simulink model "Par2_1"  (R2018a)
settings: Solver=VariableStepAuto  StartTime=0.0  StopTime=100  RelTol=1e-3
settings Model: Creator=wangluo  LastModifiedBy=wangluo

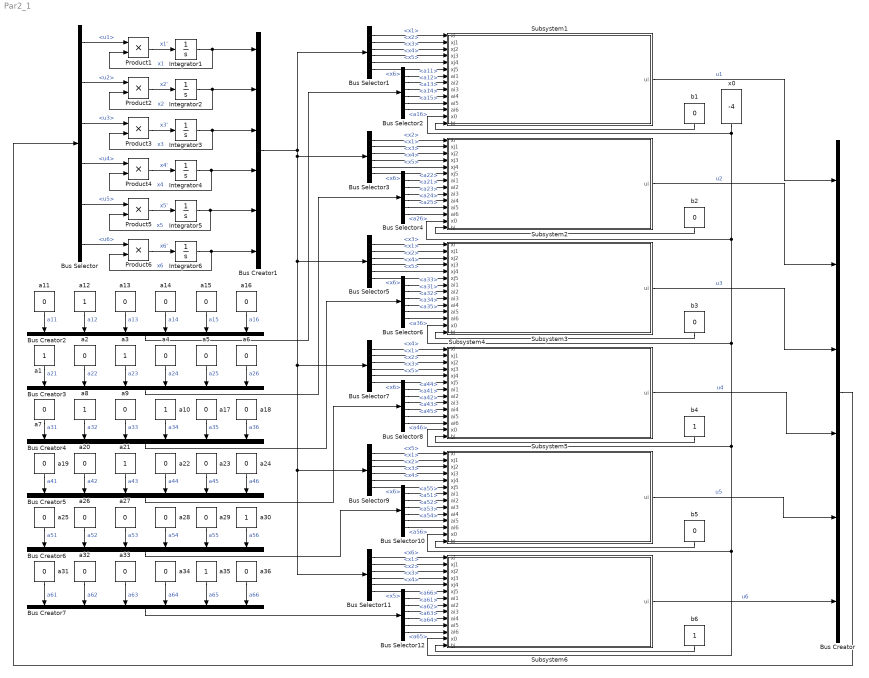
== system Par2_1 ==
  Bus Creator{,1..7} (8 alike) : BusCreator  Inputs=6
  Bus Selector : BusSelector  OutputSignals=u1,u2,u3,u4,u5,u6
  Bus Selector1 : BusSelector  OutputSignals=x1,x2,x3,x4,x5,x6
  Bus Selector10 : BusSelector  OutputSignals=a55,a51,a52,a53,a54,a56
  Bus Selector11 : BusSelector  OutputSignals=x6,x1,x2,x3,x4,x5
  Bus Selector12 : BusSelector  OutputSignals=a66,a61,a62,a63,a64,a65
  Bus Selector2 : BusSelector  OutputSignals=a11,a12,a13,a14,a15,a16
  Bus Selector3 : BusSelector  OutputSignals=x2,x1,x3,x4,x5,x6
  Bus Selector4 : BusSelector  OutputSignals=a22,a21,a23,a24,a25,a26
  Bus Selector5 : BusSelector  OutputSignals=x3,x1,x2,x4,x5,x6
  Bus Selector6 : BusSelector  OutputSignals=a33,a31,a32,a34,a35,a36
  Bus Selector7 : BusSelector  OutputSignals=x4,x1,x2,x3,x5,x6
  Bus Selector8 : BusSelector  OutputSignals=a44,a41,a42,a43,a45,a46
  Bus Selector9 : BusSelector  OutputSignals=x5,x1,x2,x3,x4,x6
  Integrator1 : Integrator  InitialCondition=1
  Integrator2 : Integrator  InitialCondition=7
  Integrator3 : Integrator  InitialCondition=0.5
  Integrator4 : Integrator  InitialCondition=5
  Integrator5 : Integrator  InitialCondition=3
  Integrator6 : Integrator  InitialCondition=8
  Product{1..6} (6 alike) : Product
  Subsystem1 : Subsystem
  Subsystem2 : Subsystem
  Subsystem3 : Subsystem
  Subsystem4 : Subsystem
  Subsystem5 : Subsystem
  Subsystem6 : Subsystem
  a{1,3,8,10,12,21,30,35} (8 alike) : Constant
  a{2,4..7,9,11,13..20,22..29,31..34,36} (28 alike) : Constant  Value=0
  b{1..3,5} (4 alike) : Constant  Value=0
  b4 : Constant
  b6 : Constant
  x0 : Constant  Value=-4
  wires:
  Integrator1/1 -> Product1/2, Bus Creator1/1  "x1"
  Integrator2/1 -> Product2/2, Bus Creator1/2  "x2"
  Bus Creator/1 -> Bus Selector/1
  Subsystem2/1(ui) -> Bus Creator/2  "u2"
  Subsystem3/1(ui) -> Bus Creator/3  "u3"
  Subsystem4/1(ui) -> Bus Creator/4  "u4"
  Subsystem5/1(ui) -> Bus Creator/5  "u5"
  Subsystem6/1(ui) -> Bus Creator/6  "u6"
  Product1/1 -> Integrator1/1  "x1'"
  Product4/1 -> Integrator4/1  "x4'"
  Product3/1 -> Integrator3/1  "x3'"
  Product2/1 -> Integrator2/1  "x2'"
  Product5/1 -> Integrator5/1  "x5'"
  Product6/1 -> Integrator6/1  "x6'"
  Integrator3/1 -> Product3/2, Bus Creator1/3  "x3"
  Integrator4/1 -> Product4/2, Bus Creator1/4  "x4"
  Integrator5/1 -> Product5/2, Bus Creator1/5  "x5"
  Integrator6/1 -> Product6/2, Bus Creator1/6  "x6"
  Bus Selector/3 -> Product3/1  "<u3>"
  Bus Selector/1 -> Product1/1  "<u1>"
  Bus Selector/2 -> Product2/1  "<u2>"
  Bus Selector/4 -> Product4/1  "<u4>"
  Bus Selector/5 -> Product5/1  "<u5>"
  Bus Selector/6 -> Product6/1  "<u6>"
  Bus Selector1/1 -> Subsystem1/1(xi)  "<x1>"
  Bus Selector1/2 -> Subsystem1/2(xj1)  "<x2>"
  Bus Selector1/3 -> Subsystem1/3(xj2)  "<x3>"
  Bus Selector1/4 -> Subsystem1/4(xj3)  "<x4>"
  Bus Selector1/5 -> Subsystem1/5(xj4)  "<x5>"
  Bus Selector1/6 -> Subsystem1/6(xj5)  "<x6>"
  Bus Creator1/1 -> Bus Selector3/1, Bus Selector5/1, Bus Selector11/1, Bus Selector9/1, Bus Selector7/1, Bus Selector1/1
  a13/1 -> Bus Creator2/3  "a13"
  a14/1 -> Bus Creator2/4  "a14"
  a11/1 -> Bus Creator2/1  "a11"
  a12/1 -> Bus Creator2/2  "a12"
  a15/1 -> Bus Creator2/5  "a15"
  a16/1 -> Bus Creator2/6  "a16"
  Bus Creator2/1 -> Bus Selector2/1
  a4/1 -> Bus Creator3/4  "a24"
  a6/1 -> Bus Creator3/6  "a26"
  Bus Creator3/1 -> Bus Selector4/1
  a5/1 -> Bus Creator3/5  "a25"
  a3/1 -> Bus Creator3/3  "a23"
  a2/1 -> Bus Creator3/2  "a22"
  a1/1 -> Bus Creator3/1  "a21"
  a10/1 -> Bus Creator4/4  "a34"
  a18/1 -> Bus Creator4/6  "a36"
  Bus Creator4/1 -> Bus Selector6/1
  a17/1 -> Bus Creator4/5  "a35"
  a9/1 -> Bus Creator4/3  "a33"
  a8/1 -> Bus Creator4/2  "a32"
  a7/1 -> Bus Creator4/1  "a31"
  a22/1 -> Bus Creator5/4  "a44"
  a24/1 -> Bus Creator5/6  "a46"
  Bus Creator5/1 -> Bus Selector8/1
  a23/1 -> Bus Creator5/5  "a45"
  a21/1 -> Bus Creator5/3  "a43"
  a20/1 -> Bus Creator5/2  "a42"
  a19/1 -> Bus Creator5/1  "a41"
  a28/1 -> Bus Creator6/4  "a54"
  a30/1 -> Bus Creator6/6  "a56"
  Bus Creator6/1 -> Bus Selector10/1
  a29/1 -> Bus Creator6/5  "a55"
  a27/1 -> Bus Creator6/3  "a53"
  a26/1 -> Bus Creator6/2  "a52"
  a25/1 -> Bus Creator6/1  "a51"
  a34/1 -> Bus Creator7/4  "a64"
  a36/1 -> Bus Creator7/6  "a66"
  Bus Creator7/1 -> Bus Selector12/1
  a35/1 -> Bus Creator7/5  "a65"
  a33/1 -> Bus Creator7/3  "a63"
  a32/1 -> Bus Creator7/2  "a62"
  a31/1 -> Bus Creator7/1  "a61"
  b1/1 -> Subsystem1/14(bi)
  b3/1 -> Subsystem3/14(bi)
  b4/1 -> Subsystem4/14(bi)
  b5/1 -> Subsystem5/14(bi)
  b6/1 -> Subsystem6/14(bi)
  x0/1 -> Subsystem2/13(x0), Subsystem3/13(x0), Subsystem6/13(x0), Subsystem5/13(x0), Subsystem4/13(x0), Subsystem1/13(x0)
  Subsystem1/1(ui) -> Bus Creator/1  "u1"
  Bus Selector3/1 -> Subsystem2/1(xi)  "<x2>"
  Bus Selector3/3 -> Subsystem2/3(xj2)  "<x3>"
  Bus Selector3/4 -> Subsystem2/4(xj3)  "<x4>"
  Bus Selector3/5 -> Subsystem2/5(xj4)  "<x5>"
  Bus Selector3/6 -> Subsystem2/6(xj5)  "<x6>"
  Bus Selector2/1 -> Subsystem1/7(ai1)  "<a11>"
  Bus Selector2/2 -> Subsystem1/8(ai2)  "<a12>"
  Bus Selector2/3 -> Subsystem1/9(ai3)  "<a13>"
  Bus Selector2/4 -> Subsystem1/10(ai4)  "<a14>"
  Bus Selector2/5 -> Subsystem1/11(ai5)  "<a15>"
  Bus Selector2/6 -> Subsystem1/12(ai6)  "<a16>"
  Bus Selector3/2 -> Subsystem2/2(xj1)  "<x1>"
  b2/1 -> Subsystem2/14(bi)
  Bus Selector5/1 -> Subsystem3/1(xi)  "<x3>"
  Bus Selector5/2 -> Subsystem3/2(xj1)  "<x1>"
  Bus Selector5/3 -> Subsystem3/3(xj2)  "<x2>"
  Bus Selector5/4 -> Subsystem3/4(xj3)  "<x4>"
  Bus Selector5/5 -> Subsystem3/5(xj4)  "<x5>"
  Bus Selector5/6 -> Subsystem3/6(xj5)  "<x6>"
  Bus Selector7/1 -> Subsystem4/1(xi)  "<x4>"
  Bus Selector7/2 -> Subsystem4/2(xj1)  "<x1>"
  Bus Selector7/3 -> Subsystem4/3(xj2)  "<x2>"
  Bus Selector7/4 -> Subsystem4/4(xj3)  "<x3>"
  Bus Selector7/5 -> Subsystem4/5(xj4)  "<x5>"
  Bus Selector7/6 -> Subsystem4/6(xj5)  "<x6>"
  Bus Selector4/1 -> Subsystem2/7(ai1)  "<a22>"
  Bus Selector4/2 -> Subsystem2/8(ai2)  "<a21>"
  Bus Selector4/3 -> Subsystem2/9(ai3)  "<a23>"
  Bus Selector4/4 -> Subsystem2/10(ai4)  "<a24>"
  Bus Selector4/5 -> Subsystem2/11(ai5)  "<a25>"
  Bus Selector4/6 -> Subsystem2/12(ai6)  "<a26>"
  Bus Selector6/1 -> Subsystem3/7(ai1)  "<a33>"
  Bus Selector6/2 -> Subsystem3/8(ai2)  "<a31>"
  Bus Selector6/3 -> Subsystem3/9(ai3)  "<a32>"
  Bus Selector6/4 -> Subsystem3/10(ai4)  "<a34>"
  Bus Selector6/5 -> Subsystem3/11(ai5)  "<a35>"
  Bus Selector6/6 -> Subsystem3/12(ai6)  "<a36>"
  Bus Selector8/1 -> Subsystem4/7(ai1)  "<a44>"
  Bus Selector8/2 -> Subsystem4/8(ai2)  "<a41>"
  Bus Selector8/3 -> Subsystem4/9(ai3)  "<a42>"
  Bus Selector8/4 -> Subsystem4/10(ai4)  "<a43>"
  Bus Selector8/5 -> Subsystem4/11(ai5)  "<a45>"
  Bus Selector8/6 -> Subsystem4/12(ai6)  "<a46>"
  Bus Selector9/1 -> Subsystem5/1(xi)  "<x5>"
  Bus Selector9/2 -> Subsystem5/2(xj1)  "<x1>"
  Bus Selector9/3 -> Subsystem5/3(xj2)  "<x2>"
  Bus Selector9/4 -> Subsystem5/4(xj3)  "<x3>"
  Bus Selector9/5 -> Subsystem5/5(xj4)  "<x4>"
  Bus Selector9/6 -> Subsystem5/6(xj5)  "<x6>"
  Bus Selector10/1 -> Subsystem5/7(ai1)  "<a55>"
  Bus Selector10/2 -> Subsystem5/8(ai2)  "<a51>"
  Bus Selector10/3 -> Subsystem5/9(ai3)  "<a52>"
  Bus Selector10/4 -> Subsystem5/10(ai4)  "<a53>"
  Bus Selector10/5 -> Subsystem5/11(ai5)  "<a54>"
  Bus Selector10/6 -> Subsystem5/12(ai6)  "<a56>"
  Bus Selector11/1 -> Subsystem6/1(xi)  "<x6>"
  Bus Selector11/2 -> Subsystem6/2(xj1)  "<x1>"
  Bus Selector11/3 -> Subsystem6/3(xj2)  "<x2>"
  Bus Selector11/4 -> Subsystem6/4(xj3)  "<x3>"
  Bus Selector11/5 -> Subsystem6/5(xj4)  "<x4>"
  Bus Selector11/6 -> Subsystem6/6(xj5)  "<x5>"
  Bus Selector12/1 -> Subsystem6/7(ai1)  "<a66>"
  Bus Selector12/2 -> Subsystem6/8(ai2)  "<a61>"
  Bus Selector12/3 -> Subsystem6/9(ai3)  "<a62>"
  Bus Selector12/4 -> Subsystem6/10(ai4)  "<a63>"
  Bus Selector12/5 -> Subsystem6/11(ai5)  "<a64>"
  Bus Selector12/6 -> Subsystem6/12(ai6)  "<a65>"

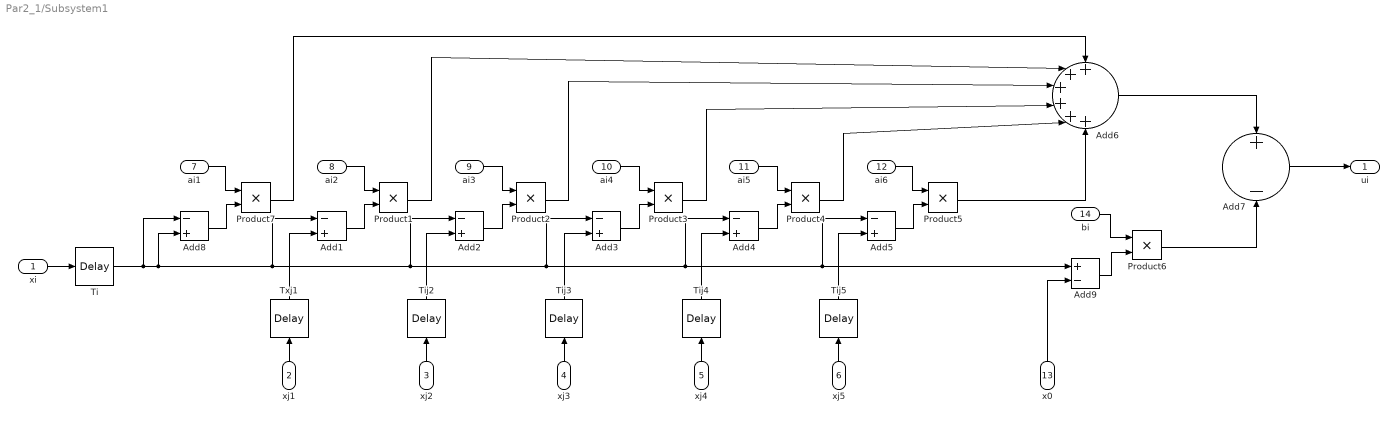
== system Par2_1/Subsystem1 ==
  xi : Inport
  xj1 : Inport  Port=2
  xj2 : Inport  Port=3
  xj3 : Inport  Port=4
  xj4 : Inport  Port=5
  xj5 : Inport  Port=6
  ai1 : Inport  Port=7
  ai2 : Inport  Port=8
  ai3 : Inport  Port=9
  ai4 : Inport  Port=10
  ai5 : Inport  Port=11
  ai6 : Inport  Port=12
  x0 : Inport  Port=13
  bi : Inport  Port=14
  Add{1..5,8} (6 alike) : Sum  Inputs=-+
  Add6 : Sum  Inputs=++++++
  Add7 : Sum  Inputs=+-
  Add9 : Sum  Inputs=+-
  Product{1..7} (7 alike) : Product
  Ti : TransportDelay  DelayTime=0
  Tij{2..5} (4 alike) : TransportDelay  DelayTime=0
  Txj1 : TransportDelay  DelayTime=0
  ui : Outport
  wires:
  Product7/1 -> Add6/1
  Add8/1 -> Product7/2
  ai1/1 -> Product7/1
  ai2/1 -> Product1/1
  Add1/1 -> Product1/2
  ai3/1 -> Product2/1
  Add2/1 -> Product2/2
  ai4/1 -> Product3/1
  Add3/1 -> Product3/2
  ai5/1 -> Product4/1
  Add4/1 -> Product4/2
  ai6/1 -> Product5/1
  Add5/1 -> Product5/2
  xi/1 -> Ti/1
  xj5/1 -> Tij5/1
  xj1/1 -> Txj1/1
  Ti/1 -> Add5/1, Add9/1, Add4/1, Add3/1, Add2/1, Add1/1, Add8/2, Add8/1
  Txj1/1 -> Add1/2
  xj2/1 -> Tij2/1
  xj3/1 -> Tij3/1
  xj4/1 -> Tij4/1
  Tij5/1 -> Add5/2
  Tij2/1 -> Add2/2
  Tij3/1 -> Add3/2
  Tij4/1 -> Add4/2
  Product5/1 -> Add6/6
  Product4/1 -> Add6/5
  Product3/1 -> Add6/4
  Product2/1 -> Add6/3
  Product1/1 -> Add6/2
  Add9/1 -> Product6/2
  bi/1 -> Product6/1
  x0/1 -> Add9/2
  Add6/1 -> Add7/1
  Product6/1 -> Add7/2
  Add7/1 -> ui/1

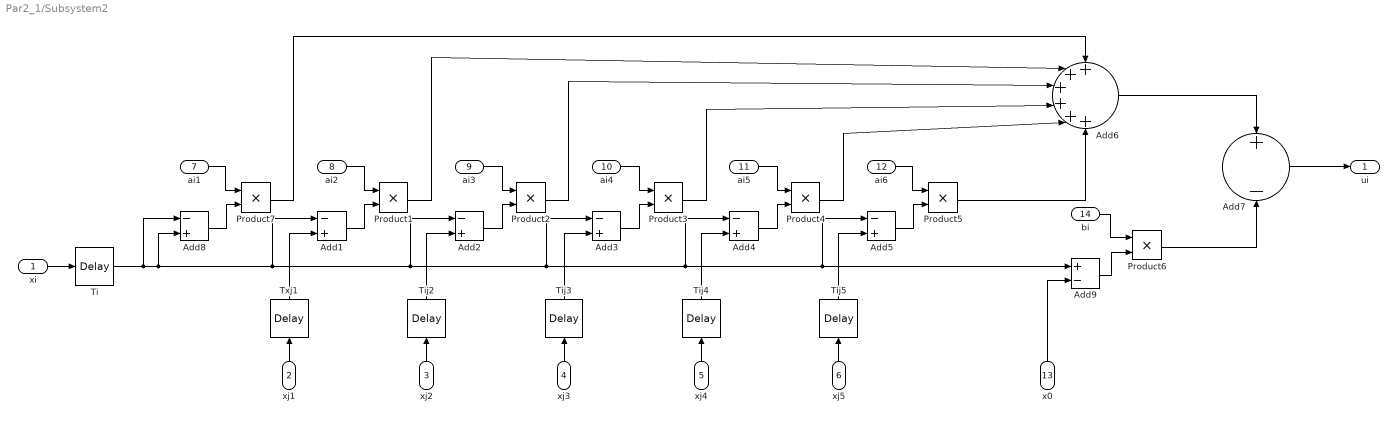
== system Par2_1/Subsystem2 ==
  xi : Inport
  xj1 : Inport  Port=2
  xj2 : Inport  Port=3
  xj3 : Inport  Port=4
  xj4 : Inport  Port=5
  xj5 : Inport  Port=6
  ai1 : Inport  Port=7
  ai2 : Inport  Port=8
  ai3 : Inport  Port=9
  ai4 : Inport  Port=10
  ai5 : Inport  Port=11
  ai6 : Inport  Port=12
  x0 : Inport  Port=13
  bi : Inport  Port=14
  Add{1..5,8} (6 alike) : Sum  Inputs=-+
  Add6 : Sum  Inputs=++++++
  Add7 : Sum  Inputs=+-
  Add9 : Sum  Inputs=+-
  Product{1..7} (7 alike) : Product
  Ti : TransportDelay  DelayTime=0
  Tij{2..5} (4 alike) : TransportDelay  DelayTime=0
  Txj1 : TransportDelay  DelayTime=0
  ui : Outport
  wires:
  Product7/1 -> Add6/1
  Add8/1 -> Product7/2
  ai1/1 -> Product7/1
  ai2/1 -> Product1/1
  Add1/1 -> Product1/2
  ai3/1 -> Product2/1
  Add2/1 -> Product2/2
  ai4/1 -> Product3/1
  Add3/1 -> Product3/2
  ai5/1 -> Product4/1
  Add4/1 -> Product4/2
  ai6/1 -> Product5/1
  Add5/1 -> Product5/2
  xi/1 -> Ti/1
  xj5/1 -> Tij5/1
  xj1/1 -> Txj1/1
  Ti/1 -> Add5/1, Add9/1, Add4/1, Add3/1, Add2/1, Add1/1, Add8/2, Add8/1
  Txj1/1 -> Add1/2
  xj2/1 -> Tij2/1
  xj3/1 -> Tij3/1
  xj4/1 -> Tij4/1
  Tij5/1 -> Add5/2
  Tij2/1 -> Add2/2
  Tij3/1 -> Add3/2
  Tij4/1 -> Add4/2
  Product5/1 -> Add6/6
  Product4/1 -> Add6/5
  Product3/1 -> Add6/4
  Product2/1 -> Add6/3
  Product1/1 -> Add6/2
  Add9/1 -> Product6/2
  bi/1 -> Product6/1
  x0/1 -> Add9/2
  Add6/1 -> Add7/1
  Product6/1 -> Add7/2
  Add7/1 -> ui/1

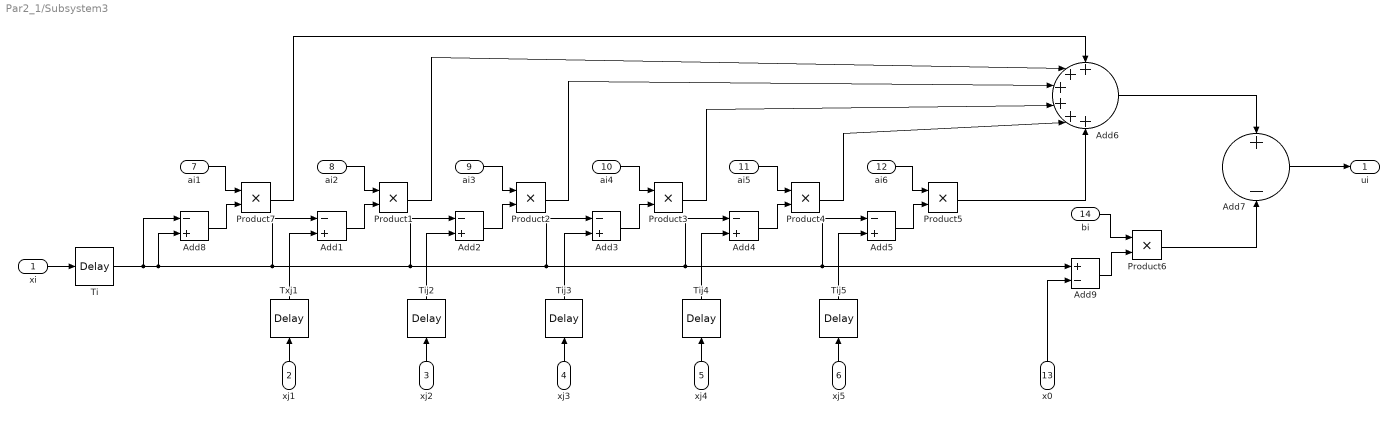
== system Par2_1/Subsystem3 ==
  xi : Inport
  xj1 : Inport  Port=2
  xj2 : Inport  Port=3
  xj3 : Inport  Port=4
  xj4 : Inport  Port=5
  xj5 : Inport  Port=6
  ai1 : Inport  Port=7
  ai2 : Inport  Port=8
  ai3 : Inport  Port=9
  ai4 : Inport  Port=10
  ai5 : Inport  Port=11
  ai6 : Inport  Port=12
  x0 : Inport  Port=13
  bi : Inport  Port=14
  Add{1..5,8} (6 alike) : Sum  Inputs=-+
  Add6 : Sum  Inputs=++++++
  Add7 : Sum  Inputs=+-
  Add9 : Sum  Inputs=+-
  Product{1..7} (7 alike) : Product
  Ti : TransportDelay  DelayTime=0
  Tij{2..5} (4 alike) : TransportDelay  DelayTime=0
  Txj1 : TransportDelay  DelayTime=0
  ui : Outport
  wires:
  Product7/1 -> Add6/1
  Add8/1 -> Product7/2
  ai1/1 -> Product7/1
  ai2/1 -> Product1/1
  Add1/1 -> Product1/2
  ai3/1 -> Product2/1
  Add2/1 -> Product2/2
  ai4/1 -> Product3/1
  Add3/1 -> Product3/2
  ai5/1 -> Product4/1
  Add4/1 -> Product4/2
  ai6/1 -> Product5/1
  Add5/1 -> Product5/2
  xi/1 -> Ti/1
  xj5/1 -> Tij5/1
  xj1/1 -> Txj1/1
  Ti/1 -> Add5/1, Add9/1, Add4/1, Add3/1, Add2/1, Add1/1, Add8/2, Add8/1
  Txj1/1 -> Add1/2
  xj2/1 -> Tij2/1
  xj3/1 -> Tij3/1
  xj4/1 -> Tij4/1
  Tij5/1 -> Add5/2
  Tij2/1 -> Add2/2
  Tij3/1 -> Add3/2
  Tij4/1 -> Add4/2
  Product5/1 -> Add6/6
  Product4/1 -> Add6/5
  Product3/1 -> Add6/4
  Product2/1 -> Add6/3
  Product1/1 -> Add6/2
  Add9/1 -> Product6/2
  bi/1 -> Product6/1
  x0/1 -> Add9/2
  Add6/1 -> Add7/1
  Product6/1 -> Add7/2
  Add7/1 -> ui/1

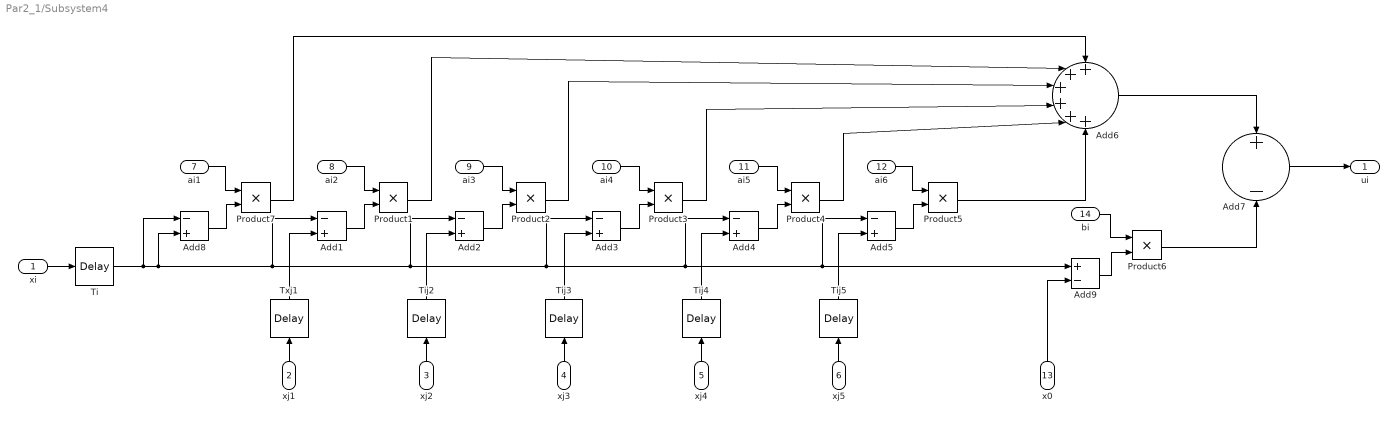
== system Par2_1/Subsystem4 ==
  xi : Inport
  xj1 : Inport  Port=2
  xj2 : Inport  Port=3
  xj3 : Inport  Port=4
  xj4 : Inport  Port=5
  xj5 : Inport  Port=6
  ai1 : Inport  Port=7
  ai2 : Inport  Port=8
  ai3 : Inport  Port=9
  ai4 : Inport  Port=10
  ai5 : Inport  Port=11
  ai6 : Inport  Port=12
  x0 : Inport  Port=13
  bi : Inport  Port=14
  Add{1..5,8} (6 alike) : Sum  Inputs=-+
  Add6 : Sum  Inputs=++++++
  Add7 : Sum  Inputs=+-
  Add9 : Sum  Inputs=+-
  Product{1..7} (7 alike) : Product
  Ti : TransportDelay  DelayTime=0
  Tij{2..5} (4 alike) : TransportDelay  DelayTime=0
  Txj1 : TransportDelay  DelayTime=0
  ui : Outport
  wires:
  Product7/1 -> Add6/1
  Add8/1 -> Product7/2
  ai1/1 -> Product7/1
  ai2/1 -> Product1/1
  Add1/1 -> Product1/2
  ai3/1 -> Product2/1
  Add2/1 -> Product2/2
  ai4/1 -> Product3/1
  Add3/1 -> Product3/2
  ai5/1 -> Product4/1
  Add4/1 -> Product4/2
  ai6/1 -> Product5/1
  Add5/1 -> Product5/2
  xi/1 -> Ti/1
  xj5/1 -> Tij5/1
  xj1/1 -> Txj1/1
  Ti/1 -> Add5/1, Add9/1, Add4/1, Add3/1, Add2/1, Add1/1, Add8/2, Add8/1
  Txj1/1 -> Add1/2
  xj2/1 -> Tij2/1
  xj3/1 -> Tij3/1
  xj4/1 -> Tij4/1
  Tij5/1 -> Add5/2
  Tij2/1 -> Add2/2
  Tij3/1 -> Add3/2
  Tij4/1 -> Add4/2
  Product5/1 -> Add6/6
  Product4/1 -> Add6/5
  Product3/1 -> Add6/4
  Product2/1 -> Add6/3
  Product1/1 -> Add6/2
  Add9/1 -> Product6/2
  bi/1 -> Product6/1
  x0/1 -> Add9/2
  Add6/1 -> Add7/1
  Product6/1 -> Add7/2
  Add7/1 -> ui/1

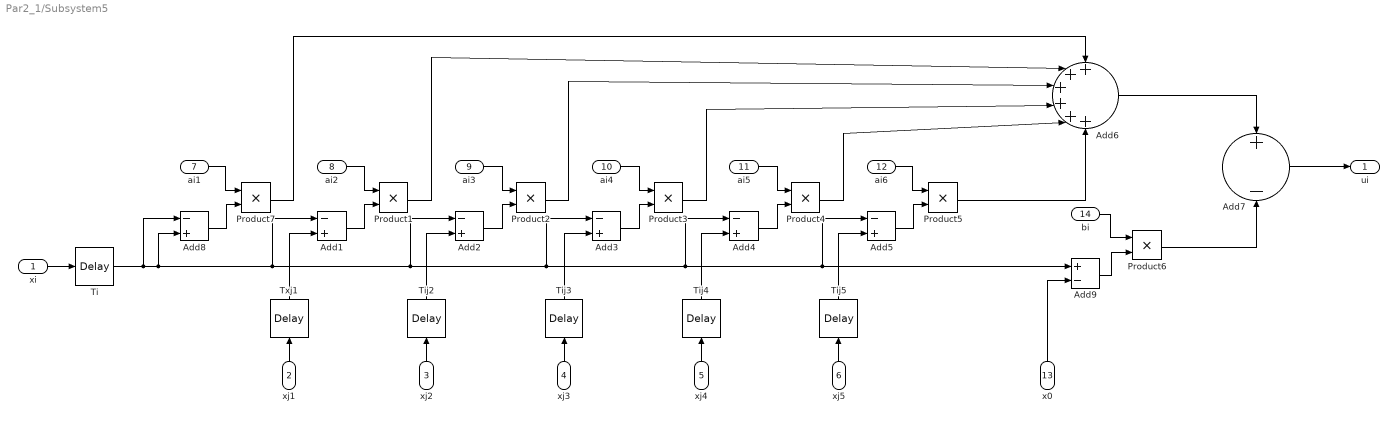
== system Par2_1/Subsystem5 ==
  xi : Inport
  xj1 : Inport  Port=2
  xj2 : Inport  Port=3
  xj3 : Inport  Port=4
  xj4 : Inport  Port=5
  xj5 : Inport  Port=6
  ai1 : Inport  Port=7
  ai2 : Inport  Port=8
  ai3 : Inport  Port=9
  ai4 : Inport  Port=10
  ai5 : Inport  Port=11
  ai6 : Inport  Port=12
  x0 : Inport  Port=13
  bi : Inport  Port=14
  Add{1..5,8} (6 alike) : Sum  Inputs=-+
  Add6 : Sum  Inputs=++++++
  Add7 : Sum  Inputs=+-
  Add9 : Sum  Inputs=+-
  Product{1..7} (7 alike) : Product
  Ti : TransportDelay  DelayTime=0
  Tij{2..5} (4 alike) : TransportDelay  DelayTime=0
  Txj1 : TransportDelay  DelayTime=0
  ui : Outport
  wires:
  Product7/1 -> Add6/1
  Add8/1 -> Product7/2
  ai1/1 -> Product7/1
  ai2/1 -> Product1/1
  Add1/1 -> Product1/2
  ai3/1 -> Product2/1
  Add2/1 -> Product2/2
  ai4/1 -> Product3/1
  Add3/1 -> Product3/2
  ai5/1 -> Product4/1
  Add4/1 -> Product4/2
  ai6/1 -> Product5/1
  Add5/1 -> Product5/2
  xi/1 -> Ti/1
  xj5/1 -> Tij5/1
  xj1/1 -> Txj1/1
  Ti/1 -> Add5/1, Add9/1, Add4/1, Add3/1, Add2/1, Add1/1, Add8/2, Add8/1
  Txj1/1 -> Add1/2
  xj2/1 -> Tij2/1
  xj3/1 -> Tij3/1
  xj4/1 -> Tij4/1
  Tij5/1 -> Add5/2
  Tij2/1 -> Add2/2
  Tij3/1 -> Add3/2
  Tij4/1 -> Add4/2
  Product5/1 -> Add6/6
  Product4/1 -> Add6/5
  Product3/1 -> Add6/4
  Product2/1 -> Add6/3
  Product1/1 -> Add6/2
  Add9/1 -> Product6/2
  bi/1 -> Product6/1
  x0/1 -> Add9/2
  Add6/1 -> Add7/1
  Product6/1 -> Add7/2
  Add7/1 -> ui/1

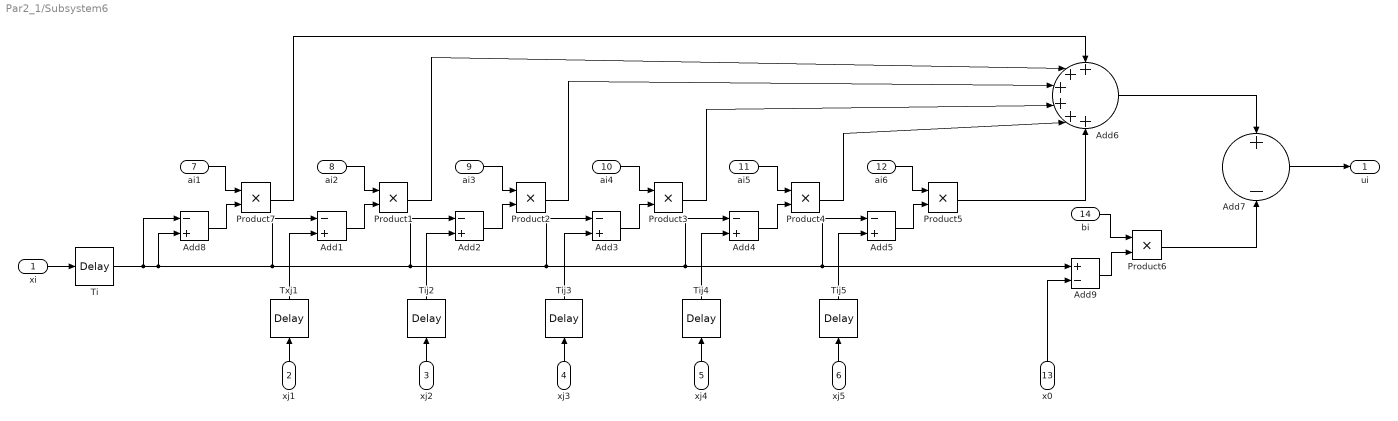
== system Par2_1/Subsystem6 ==
  xi : Inport
  xj1 : Inport  Port=2
  xj2 : Inport  Port=3
  xj3 : Inport  Port=4
  xj4 : Inport  Port=5
  xj5 : Inport  Port=6
  ai1 : Inport  Port=7
  ai2 : Inport  Port=8
  ai3 : Inport  Port=9
  ai4 : Inport  Port=10
  ai5 : Inport  Port=11
  ai6 : Inport  Port=12
  x0 : Inport  Port=13
  bi : Inport  Port=14
  Add{1..5,8} (6 alike) : Sum  Inputs=-+
  Add6 : Sum  Inputs=++++++
  Add7 : Sum  Inputs=+-
  Add9 : Sum  Inputs=+-
  Product{1..7} (7 alike) : Product
  Ti : TransportDelay  DelayTime=0
  Tij{2..5} (4 alike) : TransportDelay  DelayTime=0
  Txj1 : TransportDelay  DelayTime=0
  ui : Outport
  wires:
  Product7/1 -> Add6/1
  Add8/1 -> Product7/2
  ai1/1 -> Product7/1
  ai2/1 -> Product1/1
  Add1/1 -> Product1/2
  ai3/1 -> Product2/1
  Add2/1 -> Product2/2
  ai4/1 -> Product3/1
  Add3/1 -> Product3/2
  ai5/1 -> Product4/1
  Add4/1 -> Product4/2
  ai6/1 -> Product5/1
  Add5/1 -> Product5/2
  xi/1 -> Ti/1
  xj5/1 -> Tij5/1
  xj1/1 -> Txj1/1
  Ti/1 -> Add5/1, Add9/1, Add4/1, Add3/1, Add2/1, Add1/1, Add8/2, Add8/1
  Txj1/1 -> Add1/2
  xj2/1 -> Tij2/1
  xj3/1 -> Tij3/1
  xj4/1 -> Tij4/1
  Tij5/1 -> Add5/2
  Tij2/1 -> Add2/2
  Tij3/1 -> Add3/2
  Tij4/1 -> Add4/2
  Product5/1 -> Add6/6
  Product4/1 -> Add6/5
  Product3/1 -> Add6/4
  Product2/1 -> Add6/3
  Product1/1 -> Add6/2
  Add9/1 -> Product6/2
  bi/1 -> Product6/1
  x0/1 -> Add9/2
  Add6/1 -> Add7/1
  Product6/1 -> Add7/2
  Add7/1 -> ui/1
